simulink model "dqMPTCrealtimepara_20250223"  (R2024b)
settings: Solver=ode1  StartTime=0.0  StopTime=1  FixedStep=1e-4  RelTol=1e-3
libraries: spsDCVoltageSourceLib x1, slpidlib x1, spsPermanentMagnetSynchronousMachineLib x1, spsUniversalBridgeLib x1, sps_lib x1
settings Model: Creator=Sicong Wen  LastModifiedBy=Deng Puda
settings SolverCC: AlgebraicLoopSolver=TrustRegion
settings DebuggingCC: UnconnectedInputMsg=warning  UnconnectedOutputMsg=warning  UnconnectedLineMsg=warning
settings ModelReferenceCC: EnableRefExpFcnMdlSchedulingChecks=on
settings SFSimCC: CustomCodeUndefinedFunction=UseInterfaceOnly
settings RTWCC: GPUComputeCapability=3.5

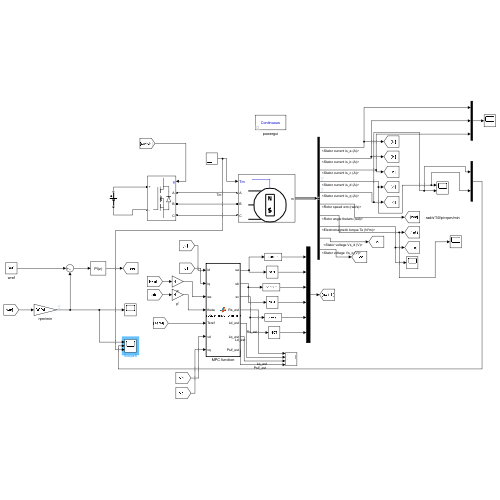
[thumbnail: Simulink's stored preview of the top-level diagram]
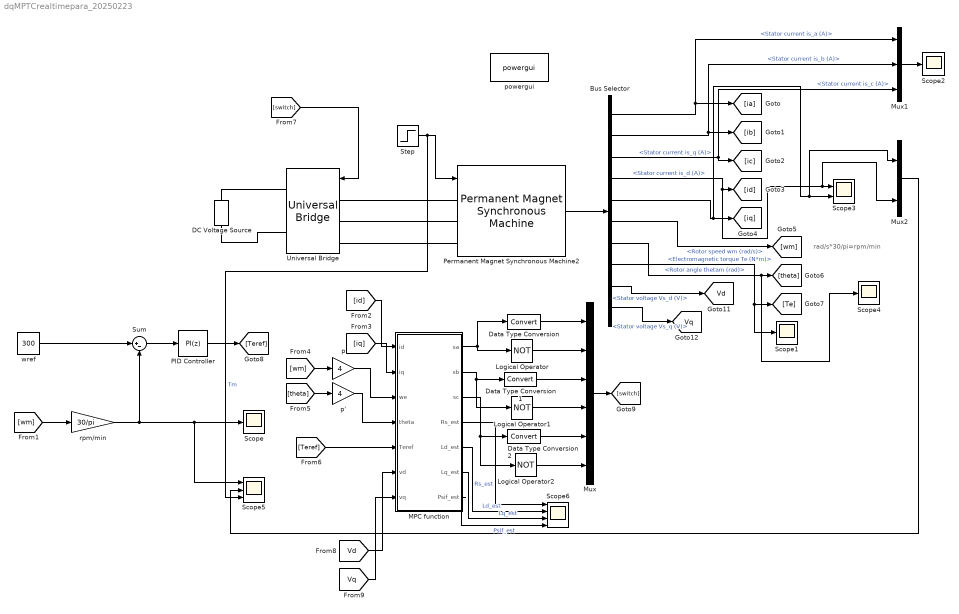
== system dqMPTCrealtimepara_20250223 ==
  note: rad/s*30/pi=rpm/min
  Bus Selector : BusSelector  OutputSignals=Stator current is_a (A),Stator current is_b (A),Stator current is_c (A),Stator current is_d (A),Stator current is_q (A),Rotor speed wm (rad/s),Rotor angle thetam (rad),Electromagnetic torque Te (N*m),Stator voltage Vs_d (V),Stator voltage Vs_q (V)
  DC Voltage Source : spsDCVoltageSourceLib/DC Voltage Source  Amplitude=48  Measurements=None
  Data Type Conversion : DataTypeConversion  SaturateOnIntegerOverflow=off  RndMeth=Floor
  Data Type Conversion1 : DataTypeConversion  SaturateOnIntegerOverflow=off  RndMeth=Floor
  Data Type Conversion2 : DataTypeConversion  SaturateOnIntegerOverflow=off  RndMeth=Floor
  Logical Operator : Logic  Operator=NOT  AllPortsSameDT=off  OutDataTypeStr=boolean
  Logical Operator1 : Logic  Operator=NOT  AllPortsSameDT=off  OutDataTypeStr=boolean
  Logical Operator2 : Logic  Operator=NOT  AllPortsSameDT=off  OutDataTypeStr=boolean
  MPC function : MATLAB Function  TreatAsAtomicUnit=on
  Mux : Mux  Inputs=6
  Mux1 : Mux  Inputs=3
  Mux2 : Mux  Inputs=2
  PID Controller : slpidlib/PID Controller  Controller=PI  Form=Parallel  TimeDomain=Discrete-time  UseExternalTs=off  SampleTime=-1  IntegratorMethod=Forward Euler  FilterMethod=Forward Euler  ControllerParametersSource=internal  P=0.5  I=5  UseKiTs=off  D=0  UseExternalDerivativeSource=off  N=100  UseFilter=on  TunerSelectOption=Transfer Function Based (PID Tuner App)  InitialConditionSource=internal  InitialConditionForIntegrator=0  InitialConditionForFilter=0  DifferentiatorICPrevScaledInput=0  ExternalReset=none  TrackingMode=off  Kt=1  LimitOutput=off  SatLimitsSource=internal  UpperSaturationLimit=inf  LowerSaturationLimit=-inf  LinearizeAsGain=on  AntiWindupMode=none  Kb=1  LimitIntegrator=off  UpperIntegratorSaturationLimit=inf  LowerIntegratorSaturationLimit=-inf  POutMin=[]  POutMax=[]  IOutMin=[]  IOutMax=[]  DOutMin=[]  DOutMax=[]  NOutMin=[]  NOutMax=[]  SumOutMin=[]  SumOutMax=[]  SaturationOutMin=[]  SaturationOutMax=[]  PParamMin=[]  PParamMax=[]  IParamMin=[]  IParamMax=[]  DParamMin=[]  DParamMax=[]  NParamMin=[]  NParamMax=[]  KbParamMin=[]  KbParamMax=[]  KtParamMin=[]  KtParamMax=[]  KbOutMin=[]  KbOutMax=[]  KtOutMin=[]  KtOutMax=[]  IntegratorOutMin=[]  IntegratorOutMax=[]  FilterOutMin=[]  FilterOutMax=[]  SumI1OutMin=[]  SumI1OutMax=[]  SumI2OutMin=[]  SumI2OutMax=[]  SumI3OutMin=[]  SumI3OutMax=[]  SumI4OutMin=[]  SumI4OutMax=[]  SumDOutMin=[]  SumDOutMax=[]  DifferentiatorOutMin=[]  DifferentiatorOutMax=[]  FilterDiffOutCoefMin=[]  FilterDiffOutCoefMax=[]  ReciprocalOutMin=[]  ReciprocalOutMax=[]  SumDenOutMin=[]  SumDenOutMax=[]  SumNumOutMin=[]  SumNumOutMax=[]  DivideOutMin=[]  DivideOutMax=[]  UdiffTsProdOutMin=[]  UdiffTsProdOutMax=[]  NTsProdOutMin=[]  NTsProdOutMax=[]  UintegralTsProdOutMin=[]  UintegralTsProdOutMax=[]  UngainTsProdOutMin=[]  UngainTsProdOutMax=[]  ClampingZeroOutDataTypeStr=Inherit: Inherit via back propagation  ClampingZeroOutMin=[]  ClampingZeroOutMax=[]  FilterDenConstantOutDataTypeStr=Inherit: Inherit via back propagation  FilterDenConstantOutMin=[]  FilterDenConstantOutMax=[]  PCopyOutDataTypeStr=Inherit: Inherit via back propagation  PCopyOutMin=[]  PCopyOutMax=[]  NCopyOutDataTypeStr=Inherit: Inherit via back propagation  NCopyOutMin=[]  NCopyOutMax=[]  IntegratorContinuousStateAttributes=''  IntegratorStateMustResolveToSignalObject=off  IntegratorRTWStateStorageClass=Auto  FilterContinuousStateAttributes=''  FilterStateMustResolveToSignalObject=off  FilterRTWStateStorageClass=Auto  ParallelPVariant=InternalParameters  IdealPVariant=Disabled  IVariant=InternalParameters  DVariant=Disabled  IntegratorVariant=Discrete  SatVariant=Disabled  AWVariant=Passthrough  PCopyVariant=Disabled  TRVariant=Disabled  FdbkBlocksVariant=Forward  IdealPFdbkVariant=Disabled  SatFdbkVariant=Disabled  DerivativeFilterVariant=Disabled  NVariant=Disabled  NCopyVariant=Disabled_SignalSpec  FilterICVariant=Disabled  IntegratorICVariant=InternalICs  ExternalResetVariant=Disabled  TRSumVariant=Passthrough  SumFdbkVariant=Disabled  SumVariant=Sum_PI  TsampFilterVariant=InternalTs  TsampNgainVariant=Passthrough  TsampIntegralVariant=Disabled_SignalSpec  ExternalSaturationOutDataTypeStr=Inherit: Same as second input  DerivativeSourceVariant=Disabled  PreIntVariant=InternalPreInt
  Permanent Magnet Synchronous Machine2 : spsPermanentMagnetSynchronousMachineLib/Permanent Magnet Synchronous Machine  NbPhases=3  FluxDistribution=Sinusoidal  RotorType=Round  MechanicalLoad=Torque Tm  PresetModel=No  ShowDetailedParameters=on  MeasurementBus=off  Resistance=1  Inductance=8.5e-3  dqInductances=[8.5e-3,8.5e-3]  La=1.4e-3  MachineConstant=Flux linkage established by magnets (V.s)  Flux=0.02  VoltageCst=14.5104  TorqueCst=0.12  Flat=120  Mechanical=[0.002 5e-3 4 0]  PolePairs=4  InitialConditions=[0,0, 0,0]  InitialConditions5ph=[0 0 0 0 0 0]  RefAngle=Aligned with phase A axis (original Park)  IterativeDiscreteModel=Trapezoidal non iterative  TsBlock=-1  TsPowergui=0
  Scope{,1..2,4} (4 alike) : Scope
  Scope3 : Scope  NumInputPorts=2
  Scope5 : Scope  NumInputPorts=3
  Scope6 : Scope  NumInputPorts=4
  Step : Step  Time=0.5  After=1.2  SampleTime=0
  Sum : Sum  Inputs=|+-
  Universal Bridge : spsUniversalBridgeLib/Universal Bridge  Arms=3  SnubberResistance=1e5  SnubberCapacitance=inf  Device=MOSFET / Diodes  Ron=1e-3  Lon=0  ForwardVoltages="[  0  0  ]"  ForwardVoltage=0  GTOparameters=[ 10e-6 , 20e-6 ]  IGBTparameters=[ 1e-6 , 2e-6 ]  Measurements=None  Measurements_2=None  converterType=Rectifier
  p : Gain  Gain=4
  p' : Gain  Gain=4
  powergui : sps_lib/powergui  Priority=1  SimulationMode=Continuous  SampleTime=1e-6  frequency=60  Iterations=50  frequencyindice=0  Pbase=100e6  ErrMax=1e-4  UnitsV=kV  UnitsW=MW  buscounter=0  FunctionMessages=off  echomessages=off  EnableUseOfTLC=off  CurrentSourceSwitches=off  DisableSnubberDevices=off  DisableRonSwitches=off  DisableVfSwitches=off  DisplayEquations=off  AutomaticDiscreteSolvers=off  SolverType=Tustin/Backward Euler (TBE)  Interpol=off  ExternalGateDelay=off  methode=off  Ts=100  x0status=blocks  SPID=on  SwTol=0  HookPort=off  NonlinearTolerance=0  nMaxIteration=15  ContinueOnMaxIteration=off  RestoreLinks=warning  ResistiveCurrentMeasurement=off  Frange=[0:2:500]  Ylog=off  Xlog=on  ShowGrid=off  save=off  variable=ZData  structure=0  ZoomFFT=off  StartTime=0.0  cycles=1  DisplayStyle=1  fundamental=60  FreqAxis=off  MaxFrequency=1000  frequencyindicesteady=1  RmsSteady=1  display=off
  rpm/min : Gain  Gain=30/pi
  wref : Constant  Value=300
  tag scope: Vd=global, Vq=global
  wires:
  Permanent Magnet Synchronous Machine2/1 -> Bus Selector/1
  Bus Selector/1 -> Mux1/1, [ia]  "<Stator current is_a (A)>"
  Bus Selector/2 -> Mux1/2, [ib]  "<Stator current is_b (A)>"
  Bus Selector/3 -> Mux1/3, [ic]  "<Stator current is_c (A)>"
  Bus Selector/5 -> Mux2/1, Scope3/2, [iq]  "<Stator current is_q (A)>"
  Bus Selector/6 -> [wm]  "<Rotor speed wm (rad/s)>"
  Bus Selector/7 -> Scope4/1, [theta]  "<Rotor angle thetam (rad)>"
  Bus Selector/8 -> Scope1/1, [Te]  "<Electromagnetic torque Te (N*m)>"
  [wm] -> rpm/min/1
  rpm/min/1 -> Scope5/1, Scope/1, Sum/2
  Sum/1 -> PID Controller/1
  PID Controller/1 -> [Teref]
  [iq] -> MPC function/2(iq)
  [id] -> MPC function/1(id)
  [wm] -> p/1
  p/1 -> MPC function/3(we)
  [theta] -> p'/1
  p'/1 -> MPC function/4(theta)
  [Teref] -> MPC function/5(Teref)
  MPC function/1(sa) -> Logical Operator/1, Data Type Conversion/1
  MPC function/2(sb) -> Logical Operator1/1, Data Type Conversion1/1
  MPC function/3(sc) -> Logical Operator2/1, Data Type Conversion2/1
  Data Type Conversion/1 -> Mux/1
  Logical Operator/1 -> Mux/2
  Data Type Conversion1/1 -> Mux/3
  Logical Operator1/1 -> Mux/4
  Data Type Conversion2/1 -> Mux/5
  Logical Operator2/1 -> Mux/6
  Mux/1 -> [switch]
  [switch] -> Universal Bridge/1
  Mux1/1 -> Scope2/1
  Step/1 -> Scope5/3, Permanent Magnet Synchronous Machine2/1  "Tm"
  Bus Selector/9 -> [Vd]  "<Stator voltage Vs_d (V)>"
  Bus Selector/10 -> [Vq]  "<Stator voltage Vs_q (V)>"
  [Vd] -> MPC function/6(vd)
  [Vq] -> MPC function/7(vq)
  MPC function/4(Rs_est) -> Scope6/1  "Rs_est"
  wref/1 -> Sum/1
  Bus Selector/4 -> Mux2/2, Scope3/1, [id]  "<Stator current is_d (A)>"
  MPC function/5(Ld_est) -> Scope6/2  "Ld_est"
  MPC function/6(Lq_est) -> Scope6/3  "Lq_est"
  MPC function/7(Psif_est) -> Scope6/4  "Psif_est"
  Mux2/1 -> Scope5/2
  connections:
  Universal Bridge/LConn1 -- Permanent Magnet Synchronous Machine2/LConn1
  Universal Bridge/LConn2 -- Permanent Magnet Synchronous Machine2/LConn2
  Universal Bridge/LConn3 -- Permanent Magnet Synchronous Machine2/LConn3
  DC Voltage Source/RConn1 -- Universal Bridge/RConn1
  DC Voltage Source/LConn1 -- Universal Bridge/RConn2

== matlab function dqMPTCrealtimepara_20250223/MPC function ==
  settings: updateMethod=DISCRETE
  data: id input; iq input; sa output; we input; theta input; Teref input; vd input; sb output; sc output; vq input; Rs_est output; Ld_est output; Lq_est output; Psif_est output
function [sa, sb, sc, Rs_est, Ld_est, Lq_est, Psif_est] = adaptive_mpc_pmsm_ekf(id, iq, we, theta, Teref, vd, vq)
    % ==========================================================
    % 终极多参数自适应 MPC 控制器 (Adaptive MPC with AEKF)
    % 解锁全部 4 个核心参数的在线预测，展示极强的鲁棒性
    % ==========================================================

    %% 1. 基础参数定义 (物理限制与系统配置)
    p = 4;                  
    vdc = 48;               % 【修改】提升到 48V，打破电压瓶颈
    Ts = 1e-4;              % 【关键修复】恢复到 10kHz，千万不能用 1e-7
    epsilon = 1e-6;         
    I_rated = 80;           

    % ==========================================================
    % 【灾难级初始猜测值】 (故意全部设错，逼迫算法去学习)
    % ==========================================================
    Rs_initial = 0.3;       % 真实值为 1.0 (相差超过3倍)
    Ld_initial = 0.8e-3;    % 真实值为 1.4e-3 (严重低估)
    Lq_initial = 0.8e-3;    % 真实值为 1.4e-3 (严重低估)
    Psif_initial = 0.01;    % 真实值为 0.02 (模拟严重的高温退磁)

    %% 2. 持久变量声明
    persistent x P Q R ifirst 
    persistent vd_prev vq_prev id_prev iq_prev we_prev
    persistent iq_ref_prev 

    %% 3. 初始化 (仅在 t=0 时运行一次)
    if isempty(ifirst)
        ifirst = 1;
        iq_ref_prev = 0;    
        
        % 状态向量 x = [Rs; Ld; Lq; Psif]
        x = [Rs_initial; Ld_initial; Lq_initial; Psif_initial];  
        
        % 初始协方差矩阵 P 
        P = diag([1e-4, 1e-6, 1e-6, 1e-6]); 
        
        % 过程噪声 Q (核心调校参数)
        Q = diag([9e-7, 1e-10, 1e-10, 1e-10]);  
        
        % 测量噪声 R
        R = diag([0.05, 0.05]); 
        
        vd_prev=0; vq_prev=0; id_prev=0; iq_prev=0; we_prev=0;
    end

    %% 4. 角度处理
    theta_elec = mod(theta, 2*pi); 

    %% 5. AEKF 核心算法 (多维状态估计)
    if ifirst == 0
        % A. 状态预测
        x_pred = x;
        P_pred = P + Q;

        % B. 计算雅可比矩阵 H (线性化预测模型)
        inv_Ld = 1 / (x(2) + epsilon);
        inv_Lq = 1 / (x(3) + epsilon);

        H = zeros(2,4);
        % 对 Rs 的偏导
        H(1,1) = -Ts * inv_Ld * id_prev;
        H(2,1) = -Ts * inv_Lq * iq_prev;
        % 对 Ld 的偏导
        H(1,2) = -Ts * (inv_Ld^2) * (vd_prev - x(1)*id_prev + we_prev*x(3)*iq_prev);
        H(2,2) = -Ts * inv_Lq * we_prev * id_prev; 
        % 对 Lq 的偏导
        H(1,3) = Ts * inv_Ld * we_prev * iq_prev;
        H(2,3) = -Ts * (inv_Lq^2) * (vq_prev - x(1)*iq_prev - we_prev*(x(2)*id_prev + x(4)));
        % 对 Psif 的偏导
        H(1,4) = 0; 
        H(2,4) = -Ts * inv_Lq * we_prev;

        % C. 计算预测电流
        id_hat = id_prev + Ts*inv_Ld*(vd_prev - x(1)*id_prev + we_prev*x(3)*iq_prev);
        iq_hat = iq_prev + Ts*inv_Lq*(vq_prev - x(1)*iq_prev - we_prev*(x(2)*id_prev + x(4)));

        % D. 测量更新 (Correction)
        y_meas = [id; iq];
        y_err = y_meas - [id_hat; iq_hat];

        S = H * P_pred * H' + R;
        K = P_pred * H' / S;

        % ==========================================================

       % 【关键：全参数自适应更新】
        x = x_pred + K * y_err;  
 
        % % 强行覆盖 EKF 的更新，制造 Fixed 模式
        % x = [0.3; 0.8e-3; 0.8e-3; 0.01];

        P = (eye(4) - K*H) * P_pred;
        % ==========================================================

        % E. 限幅保护 (极其重要：解锁所有参数，同时防止发散爆炸)
        x(1) = max(0.1, min(x(1), 2.5));       % Rs 限制
        x(2) = max(0.5e-3, min(x(2), 3.0e-3)); % Ld 限制
        x(3) = max(0.5e-3, min(x(3), 3.0e-3)); % Lq 限制
        x(4) = max(0.005, min(x(4), 0.05));    % Psif 限制

    else
        ifirst = 0; 
    end

    %% 6. 更新历史值 & 输出观测值
    Rs_est = x(1); 
    Ld_est = x(2); 
    Lq_est = x(3); 
    Psif_est = x(4); 
    
    vd_prev = vd; vq_prev = vq;
    id_prev = id; iq_prev = iq;
    we_prev = we;

    %% 7. MPC 滚动优化 (基于最新修正的精准参数)
    id_ref = 0;

    % 转矩 -> 电流参考 (使用动态更新的磁链 x(4) 才能算准 MTPA)
    iq_target = Teref / (1.5 * p * x(4)); 
    iq_target = max(-I_rated, min(I_rated, iq_target));

    % 滤波系数
    alpha = 0.8; 
    iq_ref = alpha * iq_ref_prev + (1 - alpha) * iq_target;
    iq_ref_prev = iq_ref;

    % 8矢量遍历
    vectors = [0 0 0; 0 0 1; 0 1 0; 0 1 1; 1 0 0; 1 0 1; 1 1 0; 1 1 1];
    min_cost = inf;
    optimal_index = 1;

    for k = 1:8
        s = vectors(k,:);
        % 坐标变换
        u_alpha = (2/3)*vdc * (s(1) - 0.5*s(2) - 0.5*s(3));
        u_beta  = (2/3)*vdc * (sqrt(3)/2*s(2) - sqrt(3)/2*s(3));
        ud_k = u_alpha * cos(theta_elec) + u_beta * sin(theta_elec);
        uq_k = -u_alpha * sin(theta_elec) + u_beta * cos(theta_elec);

        % 预测下一时刻 (完全使用 AEKF 吐出来的最新模型参数 x)
        id_next = id + Ts/(x(2)+epsilon) * (ud_k - x(1)*id + we*x(3)*iq);
        iq_next = iq + Ts/(x(3)+epsilon) * (uq_k - x(1)*iq - we*(x(2)*id + x(4)));

        J = (id_ref - id_next)^2 + (iq_ref - iq_next)^2;

        if J < min_cost
            min_cost = J;
            optimal_index = k;
        end
    end

    %% 8. 输出开关状态
    sa = vectors(optimal_index, 1);
    sb = vectors(optimal_index, 2);
    sc = vectors(optimal_index, 3);
end
